simulink model "DoblePendulo_MonsivasVelezJosueAdan"  (R2024a)
settings: Solver=VariableStepAuto  StartTime=0.0  StopTime=10.0  RelTol=1e-3
values from neighbouring files (symbols this model uses):
  g = 9.81    [ParametrosAct1_MonsivaisVelezJosueAdan.m]
  l1 = 0.1    [ParametrosAct1_MonsivaisVelezJosueAdan.m]
  l2 = 0.25    [ParametrosAct1_MonsivaisVelezJosueAdan.m]
  m1 = 0.2    [ParametrosAct1_MonsivaisVelezJosueAdan.m]
  m2 = 0.3    [ParametrosAct1_MonsivaisVelezJosueAdan.m]
settings Model: Creator=Dell
settings RTWCC: GPUComputeCapability=3.5

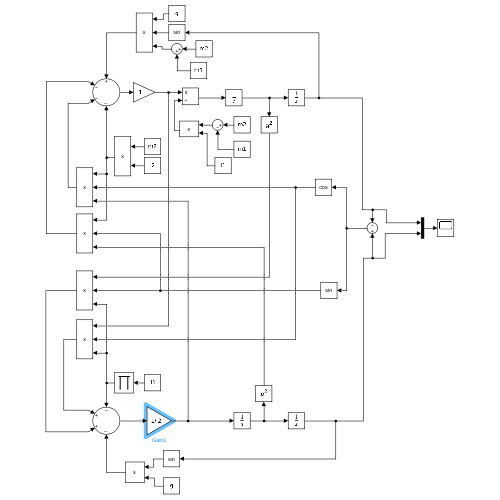
[thumbnail: Simulink's stored preview of the top-level diagram]
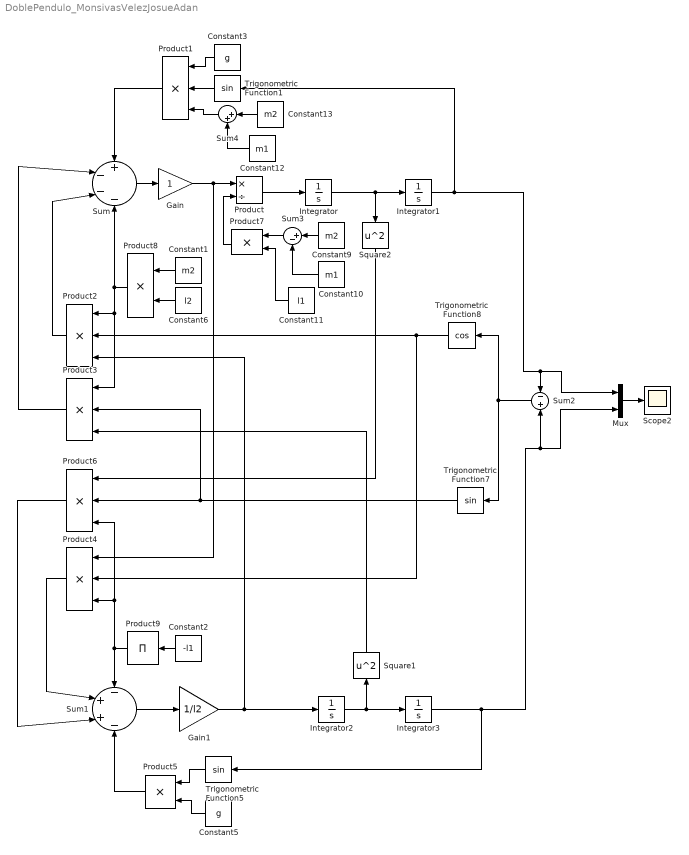
== system DoblePendulo_MonsivasVelezJosueAdan ==
  Constant1 : Constant  Value=m2
  Constant10 : Constant  Value=m1
  Constant11 : Constant  Value=l1
  Constant12 : Constant  Value=m1
  Constant13 : Constant  Value=m2
  Constant2 : Constant  Value=-l1
  Constant3 : Constant  Value=g
  Constant5 : Constant  Value=g
  Constant6 : Constant  Value=l2
  Constant9 : Constant  Value=m2
  Gain : Gain
  Gain1 : Gain  Gain=1/l2
  Integrator : Integrator
  Integrator1 : Integrator
  Integrator2 : Integrator
  Integrator3 : Integrator  InitialCondition=35*pi/180
  Mux : Mux  Inputs=2
  Product : Product  Inputs=*/
  Product{1..4,6} (5 alike) : Product  Inputs=3
  Product5 : Product
  Product7 : Product
  Product8 : Product
  Product9 : Product  Inputs=1
  Scope2 : Scope
  Square1 : Math  Operator=square  SignedPower=on  RndMeth=Zero
  Square2 : Math  Operator=square  SignedPower=on  RndMeth=Zero
  Sum : Sum  Inputs=+---
  Sum1 : Sum  Inputs=-++-
  Sum2 : Sum  Inputs=-+
  Sum3 : Sum  Inputs=|+-
  Sum4 : Sum  Inputs=|++
  Trigonometric Function1 : Trigonometry
  Trigonometric Function5 : Trigonometry
  Trigonometric Function7 : Trigonometry
  Trigonometric Function8 : Trigonometry  Operator=cos
  wires:
  Sum/1 -> Gain/1
  Gain/1 -> Product/1, Product4/1
  Integrator1/1 -> Trigonometric Function1/1, Mux/1, Sum2/1
  Sum1/1 -> Gain1/1
  Integrator/1 -> Integrator1/1, Square2/1
  Integrator3/1 -> Trigonometric Function5/1, Sum2/2, Mux/2
  Integrator2/1 -> Integrator3/1, Square1/1
  Square1/1 -> Product3/3
  Product3/1 -> Sum/2
  Product2/1 -> Sum/3
  Product1/1 -> Sum/1
  Sum4/1 -> Product1/3
  Trigonometric Function1/1 -> Product1/2
  Constant3/1 -> Product1/1
  Constant2/1 -> Product9/1
  Trigonometric Function8/1 -> Product2/2, Product4/2
  Constant5/1 -> Product5/2
  Trigonometric Function5/1 -> Product5/1
  Square2/1 -> Product6/1
  Mux/1 -> Scope2/1
  Sum2/1 -> Trigonometric Function8/1, Trigonometric Function7/1
  Trigonometric Function7/1 -> Product3/2, Product6/2
  Product/1 -> Integrator/1
  Sum3/1 -> Product7/1
  Constant10/1 -> Sum3/2
  Constant9/1 -> Sum3/1
  Constant11/1 -> Product7/2
  Product7/1 -> Product/2
  Constant12/1 -> Sum4/2
  Constant13/1 -> Sum4/1
  Product8/1 -> Sum/4, Product3/1, Product2/1
  Constant1/1 -> Product8/1
  Constant6/1 -> Product8/2
  Product5/1 -> Sum1/4
  Product9/1 -> Product6/3, Product4/3, Sum1/1
  Product4/1 -> Sum1/2
  Product6/1 -> Sum1/3
  Gain1/1 -> Integrator2/1, Product2/3
